simulink model "uloha2_6_ABS_library"  (R2020b)
settings: Solver=VariableStepAuto  StartTime=0.0  StopTime=10  RelTol=1e-3  EnableMultiTasking=on
undefined symbols (not defined in the file or in its folder): g, J, m, mi, r, skluz, v0
libraries: lib_ABS x1
settings Model: Creator=Jirkovsk  LastModifiedBy=jirkovsky
settings DataIOCC: LimitDataPoints=on  SaveFormat=Array  ReturnWorkspaceOutputs=off
settings OptimizationCC: ExpressionDepthLimit=2147483647  LifeSpan=inf
settings DebuggingCC: UnderspecifiedInitializationDetection=Classic  MergeDetectMultiDrivingBlocksExec=none  SolverPrmCheckMsg=warning  StateNameClashWarn=warning  SFUnexpectedBacktrackingDiag=warning  SFNoUnconditionalDefaultTransitionDiag=warning  SFExecutionAtInitializationDiag=none  ArithmeticOperatorsInVariantConditions=warning
settings HardwareCC: ProdBitPerPointer=32  ProdBitPerSizeT=32  ProdBitPerPtrDiffT=32  ProdLargestAtomicFloat=None  ProdIntDivRoundTo=Undefined  ProdEndianess=Unspecified  ProdWordSize=32  ProdHWDeviceType=32-bit Generic
settings ModelReferenceCC: PropagateSignalLabelsOutOfModel=off
settings SFSimCC: SimUseLocalCustomCode=off  CustomCodeUndefinedFunction=UseInterfaceOnly
settings RTWCC: RTWUseLocalCustomCode=off
settings CodeAppCC: StateflowObjectComments=on
settings GRTTargetCC: TargetLangStandard=C89/C90 (ANSI)
settings ConfigComp: CovMetricSettings=dw  CovSaveCumulativeToWorkspaceVar=on  CovSaveSingleToWorkspaceVar=on  CovExternalEMLEnable=off

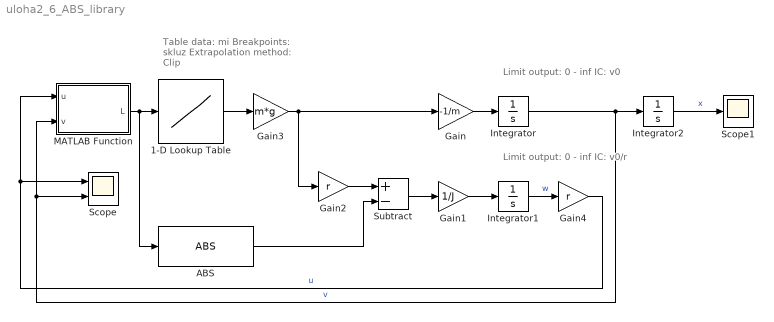
== system uloha2_6_ABS_library ==
  note: Table data: mi
      | Breakpoints: skluz
      | Extrapolation method: Clip
  note: Limit output: 0 - inf
      | IC: v0/r
  note: Limit output: 0 - inf
      | IC: v0
  1-D Lookup Table : Lookup_n-D  NumberOfTableDimensions=1  BreakpointsForDimension1=skluz  Table=mi  ExtrapMethod=Clip  RndMeth=Simplest  InputSameDT=on
  ABS : lib_ABS/ABS  wL=0.19
  Gain : Gain  Gain=-1/m
  Gain1 : Gain  Gain=1/J
  Gain2 : Gain  Gain=r
  Gain3 : Gain  Gain=m*g
  Gain4 : Gain  Gain=r
  Integrator : Integrator  InitialCondition=v0  LimitOutput=on  LowerSaturationLimit=0
  Integrator1 : Integrator  InitialCondition=v0/r  LimitOutput=on  LowerSaturationLimit=0
  Integrator2 : Integrator
  MATLAB Function : MATLAB Function  TreatAsAtomicUnit=on
  Scope : Scope  NumInputPorts=2
  Scope1 : Scope
  Subtract : Sum  Inputs=+-
  wires:
  Gain3/1 -> Gain/1, Gain2/1
  Gain/1 -> Integrator/1
  Gain1/1 -> Integrator1/1
  Subtract/1 -> Gain1/1
  Gain2/1 -> Subtract/1
  1-D Lookup Table/1 -> Gain3/1
  MATLAB Function/1(L) -> ABS/1, 1-D Lookup Table/1
  Integrator/1 -> MATLAB Function/2(v), Scope/2, Integrator2/1  "v"
  Integrator1/1 -> Gain4/1  "w"
  ABS/1 -> Subtract/2
  Integrator2/1 -> Scope1/1  "x"
  Gain4/1 -> MATLAB Function/1(u), Scope/1  "u"

== matlab function uloha2_6_ABS_library/MATLAB Function ==
  data: u input; L output; v input
function L = fcn(u,v)

L = 1 - u/v;
